simulink model "mic_controller"  (Simulink 5.0)
settings: Solver=ode45  SolverMode=SingleTasking  StartTime=0.0  StopTime=0.018  FixedStep=0.001  RelTol=1e-3
settings Model: LastModifiedBy=SHMULIK  RTWOptions="-aEnforceIntegerDowncast=1 -aFoldNonRolledExpr=1 -aInlineInvariantSignals=1 -aInlineParameters=0 -aLocalBlockOutputs=1 -aRollThreshold=5 -aZeroInternalMemoryAtStartup=1 -aZeroExternalMemoryAtStartup=1 -aInitFltsAndDblsToZero=1 -aGenerateReport=0 -aGenCodeOnly=0 -aRTWVerbose=1 -aIncludeHyperlinkInReport=0 -aLaunchReport=0 -aForceParamTrailComments=0 -aGenerateComments=1 -aIgnoreCustomStorageClasses=1 -aIncHierarchyInIds=0 -aMaxRTWIdLen=31 -aShowEliminatedStatements=0 -aPrefixModelToSubsysFcnNames=1 -aIncDataTypeInIds=0 -aInsertBlockDesc=0 -aSimulinkBlockComments=1 -aInlinedPrmAccess=\"Literals\"  -aSuppressErrorStatus=0 -aModelReferenceCompliant=0 -aSupportNonInlinedSFcns=1 -aSupportContinuousTime=1 -aSupportComplex=1 -aSupportNonFinite=1 -aSupportAbsoluteTime=1 -aTargetFcnLib=\"ansi_tfl_tmw.mat\" -aMultiInstanceERTCode=0 -aLogVarNameModifier=\"rt_\" -aIsPILTarget=0 -aCombineOutputUpdateFcns=0 -aGenerateSampleERTMain=0 -aGenerateFullHeader=1 -aUtilityFuncGeneration=\"Auto\" -aIncludeFileDelimiter=\"Auto\" -aIncludeMdlTerminateFcn=1 -aPurelyIntegerCode=0 -aERTCustomFileBanners=0 -aMatFileLogging=0 -aGenFloatMathFcnCalls=\"ANSI_C\"  -aInitFltsAndDblsToZero=1 -aGenerateASAP2=0 -aRTWCAPIStates=0 -aRTWCAPIParams=0 -aRTWCAPISignals=0 -aExtModeMexFile=\"ext_comm\" -aExtModeTransport=0 -aExtModeStaticAllocSize=1000000 -aExtModeTesting=0 -aExtModeStaticAlloc=0 -aExtMode=0"

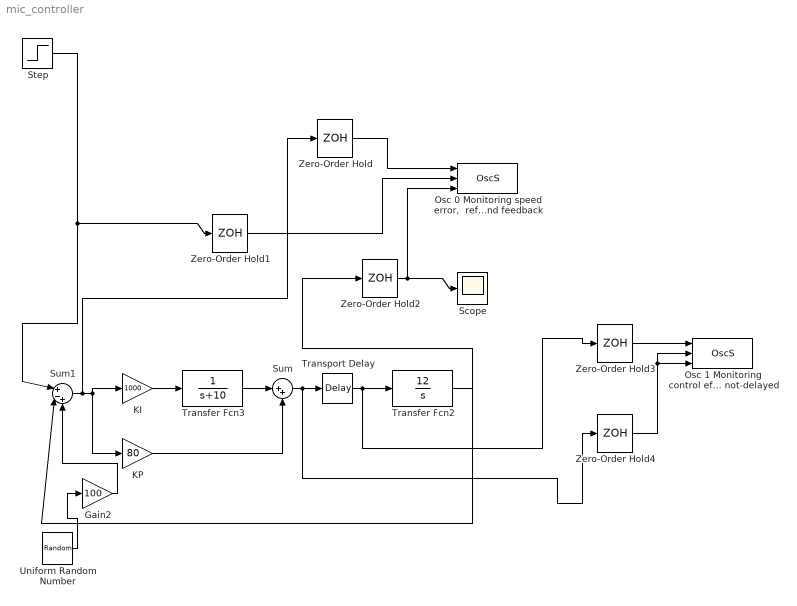
== system mic_controller ==
  Gain2 : Gain  Gain=100  SaturateOnIntegerOverflow=on
  KI : Gain  Gain=1000  SaturateOnIntegerOverflow=on
  KP : Gain  Gain=80  SaturateOnIntegerOverflow=on
  "Osc 0 Monitoring speed error,  reference and feedback" : S-Function  FunctionName=OscS  Parameters=0 , ModelScopeIniFileName , ModelScopeReload,ModelScopeClearBuffer
  Osc 1 Monitoring control effort  delayed and not-delayed : S-Function  FunctionName=OscS  Parameters="1,  ModelScopeIniFileName, ModelScopeReload,ModelScopeClearBuffer"
  Scope : Scope
  Step : Step  Time=100  Before=100  After=0  SampleTime=0
  Sum : Sum  Inputs=|++  SaturateOnIntegerOverflow=on
  Sum1 : Sum  Inputs=|+-+  SaturateOnIntegerOverflow=on
  Transfer Fcn2 : TransferFcn  Numerator=12  Denominator=[1 0]
  Transfer Fcn3 : TransferFcn  Numerator=1  Denominator="[1  10]"
  Transport Delay : TransportDelay  DelayTime=1000e-6
  Uniform Random Number : UniformRandomNumber  Minimum=-0.1  Maximum=0.1  SampleTime=0
  Zero-Order Hold{,1..4} (5 alike) : ZeroOrderHold  SampleTime=90e-6
  wires:
  Step/1 -> Sum1/1, Zero-Order Hold1/1
  Zero-Order Hold1/1 -> "Osc 0 Monitoring speed error,  reference and feedback"/2
  KI/1 -> Transfer Fcn3/1
  Transfer Fcn3/1 -> Sum/1
  KP/1 -> Sum/2
  Sum1/1 -> KI/1, KP/1, Zero-Order Hold/1
  Transfer Fcn2/1 -> Sum1/2, Zero-Order Hold2/1
  Zero-Order Hold2/1 -> "Osc 0 Monitoring speed error,  reference and feedback"/3, Scope/1
  Zero-Order Hold/1 -> "Osc 0 Monitoring speed error,  reference and feedback"/1
  Uniform Random Number/1 -> Gain2/1
  Gain2/1 -> Sum1/3
  Sum/1 -> Transport Delay/1, Zero-Order Hold4/1
  Transport Delay/1 -> Transfer Fcn2/1, Zero-Order Hold3/1
  Zero-Order Hold3/1 -> Osc 1 Monitoring control effort  delayed and not-delayed/1
  Zero-Order Hold4/1 -> Osc 1 Monitoring control effort  delayed and not-delayed/3, Osc 1 Monitoring control effort  delayed and not-delayed/2
